simulink model "rl"  (R2022b)
settings: Solver=FixedStepAuto  StartTime=0.0  StopTime=200  RelTol=1e-3
undefined symbols (not defined in the file or in its folder): a, A, b, DiscIntNeverNeededParam, Ts
libraries: rllib x1
settings Model: Creator=enes  LastModifiedBy=enes
settings SFSimCC: SimTargetLang=C++

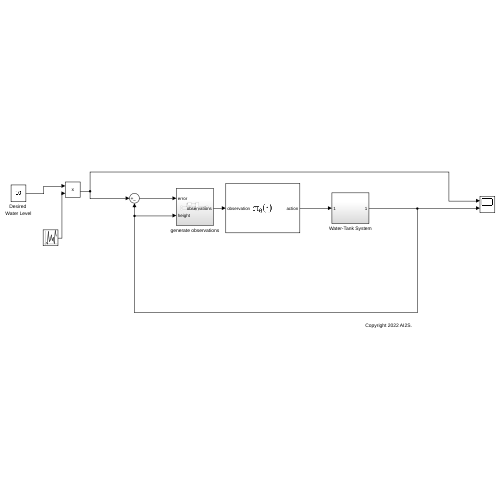
[thumbnail: Simulink's stored preview of the top-level diagram]
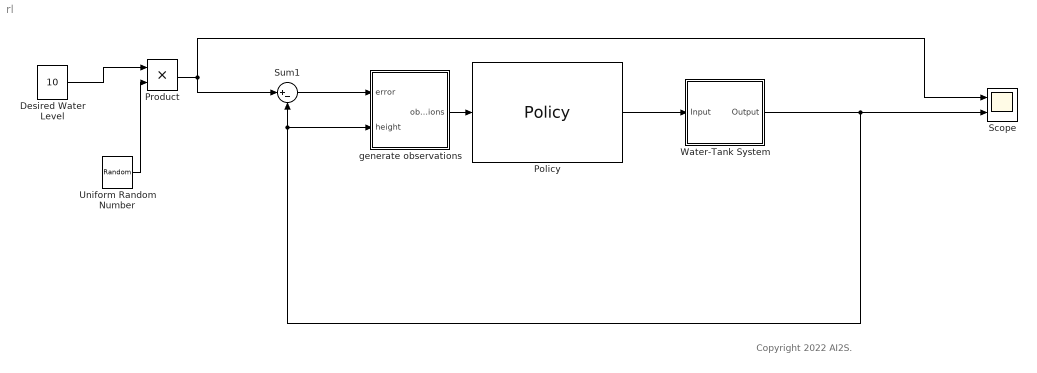
== system rl ==
  note: Copyright 2022 AI2S.
  Desired Water Level : Constant  Value=10
  Policy : rllib/Policy  MATFile=blockAgentData.mat  SimUsingCodegen=off
  Product : Product
  Scope : Scope  NumInputPorts=2
  Sum1 : Sum  Inputs=|+-  SaturateOnIntegerOverflow=on
  Uniform Random Number : UniformRandomNumber  Minimum=0  Maximum=1.5  SampleTime=25
  Water-Tank System : Subsystem
  generate observations : Subsystem
  wires:
  Desired Water Level/1 -> Product/1
  Uniform Random Number/1 -> Product/2
  Water-Tank System/1(Output) -> Scope/2, generate observations/2(height), Sum1/2
  Product/1 -> Sum1/1, Scope/1
  generate observations/1(observations) -> Policy/1
  Policy/1 -> Water-Tank System/1(Input)
  Sum1/1 -> generate observations/1(error)

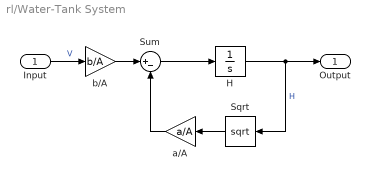
== system rl/Water-Tank System ==
  Input : Inport
  H : Integrator  LimitOutput=on  LowerSaturationLimit=0
  Sqrt : Sqrt  OutputSignalType=real
  Sum : Sum  Inputs=|+-  SaturateOnIntegerOverflow=on
  a/A : Gain  Gain=a/A  SaturateOnIntegerOverflow=on  OutDataTypeStr=Inherit: Same as input  ParamDataTypeStr=Inherit: Same as input
  b/A : Gain  Gain=b/A  SaturateOnIntegerOverflow=on  OutDataTypeStr=Inherit: Same as input  ParamDataTypeStr=Inherit: Same as input
  Output : Outport  VectorParamsAs1DForOutWhenUnconnected=off
  wires:
  b/A/1 -> Sum/1
  Sum/1 -> H/1
  H/1 -> Sqrt/1, Output/1  "H"
  Sqrt/1 -> a/A/1
  a/A/1 -> Sum/2
  Input/1 -> b/A/1  "V"

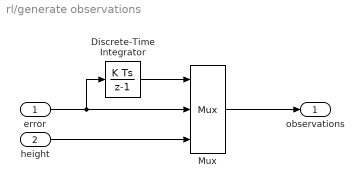
== system rl/generate observations ==
  error : Inport
  height : Inport  Port=2
  Discrete-Time Integrator : DiscreteIntegrator  SampleTime=Ts  ICPrevOutput=DiscIntNeverNeededParam  ICPrevScaledInput=DiscIntNeverNeededParam
  Mux : Mux  Inputs=3
  observations : Outport  VectorParamsAs1DForOutWhenUnconnected=off
  wires:
  height/1 -> Mux/3
  Discrete-Time Integrator/1 -> Mux/1
  error/1 -> Discrete-Time Integrator/1, Mux/2
  Mux/1 -> observations/1
